simulink model "lev2coilsZpid"  (R2022a)
settings: Solver=ode3  StartTime=0.0  StopTime=5  FixedStep=1e-3  RelTol=1e-3
values from neighbouring files (symbols this model uses):
  g = s(1:n,n+1:n+nb)    [MagLev.m]    (also in MagLev4coils.m = 9.8)
  K3 = K1    (= 5.40205233157e-05)    [MagLev4coils.m]
  K4 = K2    (= 5.40205233157e-05)    [MagLev4coils.m]
  l = 0.0567/2    (= 0.02835)    [MagLev4coils.m]
  L1 = L    (= 0.00388)    [MagLev4coils.m]
  L2 = L    (= 0.00388)    [MagLev4coils.m]
  m = 0.03    [MagLev.m]    (also in MagLev4coils.m = 0.01)
  R1 = R    (= 4)    [MagLev4coils.m]
  R2 = R    (= 4)    [MagLev4coils.m]
settings Model: Creator=macbook_pro  LastModifiedBy=macbook_pro
settings DebuggingCC: UnconnectedInputMsg=warning  UnconnectedOutputMsg=warning  UnconnectedLineMsg=warning
settings RTWCC: DLArmComputeVersion=19.05

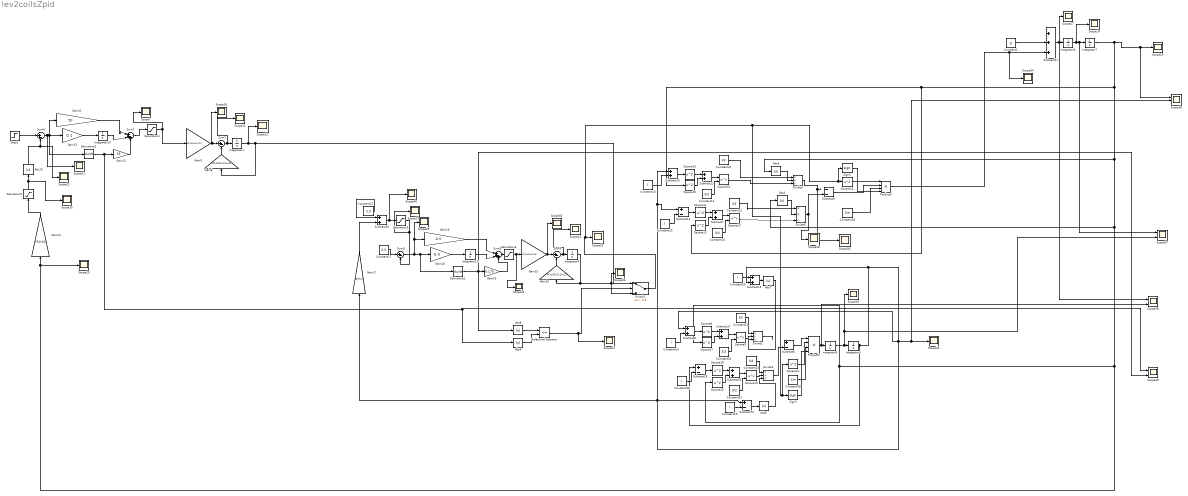
== system lev2coilsZpid ==
  Abs{4..10} (7 alike) : Abs  SaturateOnIntegerOverflow=off
  Constant1 : Constant  Value=g
  Constant11 : Constant  Value=K3
  Constant12 : Constant  Value=K4
  Constant{13,15,19..20,24,36} (6 alike) : Constant  Value=l
  Constant{14,16,34,37} (4 alike) : Constant  Value=3/2
  Constant17 : Constant  Value=2.5
  Constant18 : Constant  Value=1/m
  Constant21 : Constant  Value=K3
  Constant22 : Constant  Value=2.5
  Constant23 : Constant  Value=K4
  Constant38 : Constant  Value=1/m
  Derivative1 : Derivative
  Derivative2 : Derivative
  Divide1 : Product  Inputs=*/*
  Divide4 : Product  Inputs=*/*
  Divide5 : Product  Inputs=**/
  Divide6 : Product  Inputs=**/
  Gain10 : Gain  Gain=(R1+R2)/(L1+L2)
  Gain11 : Gain  Gain=50
  Gain12 : Gain  Gain=55
  Gain13 : Gain  Gain=0.1
  Gain14 : Gain  Gain=(5/0.04)
  Gain15 : Gain  Gain=12/((L2+L1)*5)
  Gain16 : Gain  Gain=0.175
  Gain17 : Gain  Gain=5/(l*2)
  Gain18 : Gain  Gain=0.5
  Gain19 : Gain  Gain=-0.5
  Gain8 : Gain  Gain=(R1+R2)/(L1+L2)
  Gain9 : Gain  Gain=12/((L2+L1)*5)
  Integrator{1,4,6,9..11} (6 alike) : Integrator
  Integrator5 : Integrator  InitialCondition=l
  Integrator7 : Integrator  InitialCondition=-0.03
  Product2 : Product  Inputs=4
  Product3 : Product  Inputs=4
  Relational Operator : RelationalOperator  Operator=<=  OutDataTypeStr=boolean  RndMeth=Simplest  InputSameDT=off
  Saturation3 : Saturate  UpperLimit=5  LowerLimit=0
  Saturation4 : Saturate  UpperLimit=5  LowerLimit=-5
  Saturation5 : Saturate  UpperLimit=0  LowerLimit=-5
  Saturation6 : Saturate  UpperLimit=5  LowerLimit=-5
  Scope{7,11..12,14,16..17,19..35,40..41} (25 alike) : Scope
  Scope36 : Scope  NumInputPorts=3
  Scope37 : Scope  NumInputPorts=2
  Scope38 : Scope  NumInputPorts=2
  Scope39 : Scope  NumInputPorts=2
  Sign2 : Signum
  Sign3 : Signum
  Square{8,10..11,13..15,17..18,20..21} (10 alike) : Math  Operator=square
  Square{9,12,16,19} (4 alike) : Math  Operator=pow
  Step1 : Step  Time=0  After=3.5  SampleTime=0
  Subtract{7..8,10,12,15..17,26} (8 alike) : Sum
  Subtract11 : Sum  Inputs=+++
  Subtract{6,13..14,18} (4 alike) : Sum  Inputs=+-
  Subtract9 : Sum  Inputs=--
  Sum{2..3,5..6} (4 alike) : Sum  Inputs=|+-
  Sum7 : Sum  Inputs=|+++
  Sum8 : Sum  Inputs=|+++
  Switch1 : Switch  Criteria=u2 > Threshold  Threshold=0.5  SaturateOnIntegerOverflow=off  InputSameDT=off
  wires:
  Gain8/1 -> Sum2/2
  Square9/1 -> Divide1/2
  Gain14/1 -> Saturation5/1
  Abs7/1 -> Divide1/3
  Constant19/1 -> Subtract14/2
  Gain9/1 -> Scope16/1, Sum2/1
  Abs6/1 -> Divide4/3
  Square18/1 -> Subtract26/1
  Sum7/1 -> Saturation4/1
  Constant13/1 -> Subtract10/2
  Subtract18/1 -> Square18/1
  Subtract11/1 -> Scope38/1, Scope17/1, Integrator6/1
  Sign3/1 -> Product2/4
  Square10/1 -> Subtract12/2
  Square13/1 -> Subtract7/2
  Constant36/1 -> Subtract18/2
  Step1/1 -> Sum6/1
  Square8/1 -> Subtract17/1
  Saturation4/1 -> Scope7/1, Gain9/1
  Divide1/1 -> ?
  Square16/1 -> Divide5/3
  Divide5/1 -> Scope30/1
  Divide4/1 -> Subtract6/2
  Abs4/1 -> Divide6/2
  Constant38/1 -> Product2/3
  Derivative2/1 -> Gain12/1, Abs9/1, Scope39/1
  Constant1/1 -> Subtract11/2
  Abs5/1 -> Divide5/2
  Constant12/1 -> Divide6/1
  Square11/1 -> Subtract7/1
  Sum3/1 -> Integrator4/1, Scope24/1
  Subtract12/1 -> Square16/1
  Switch1/1 -> Scope31/1, Square21/1, Sign3/1, Sign2/1, Square14/1
  Constant15/1 -> Subtract13/2
  Constant20/1 -> Subtract15/1
  Gain12/1 -> Sum7/3
  Subtract7/1 -> Square12/1
  Constant18/1 -> Product3/3
  Derivative1/1 -> Abs8/1, Gain16/1, Scope39/2
  Abs8/1 -> Relational Operator/1
  Constant37/1 -> Square19/2
  Integrator5/1 -> Subtract15/2, Subtract10/1, Subtract13/1, Gain17/1, Subtract14/1, Subtract8/1, Scope36/2, Scope23/1, Subtract18/1
  Integrator4/1 -> Scope26/1, Switch1/3, Gain10/1
  Abs9/1 -> Relational Operator/2
  Square21/1 -> Product2/2
  Product3/1 -> Scope34/1, Subtract11/3
  Subtract17/1 -> Square9/1
  Subtract26/1 -> Square19/1
  Subtract13/1 -> Square11/1
  Gain13/1 -> Integrator10/1
  Subtract15/1 -> Abs7/1
  Square20/1 -> Subtract26/2
  Gain15/1 -> Scope33/1, Sum3/1
  Integrator1/1 -> Scope12/1, Switch1/1, Gain8/1
  Integrator6/1 -> Scope37/1, Integrator7/1, Scope14/1
  Square12/1 -> Divide6/3
  Sum2/1 -> Scope11/1, Integrator1/1
  Square19/1 -> Divide4/2
  Subtract9/1 -> Product3/2
  Gain11/1 -> Sum7/1
  Abs10/1 -> Scope22/1, Sum6/2
  Sum6/1 -> Scope21/1, Derivative2/1, Gain13/1, Gain11/1
  Saturation5/1 -> Abs10/1, Scope35/1
  Sum8/1 -> Saturation6/1
  Subtract10/1 -> Square15/1
  Constant21/1 -> Divide5/1
  Square15/1 -> Subtract12/1
  Product2/1 -> Scope38/2, Integrator9/1
  Sum5/1 -> Gain19/1, Scope25/1, Derivative1/1, Gain18/1
  Gain18/1 -> Integrator11/1
  Divide6/1 -> Scope28/1, Subtract9/2
  Subtract8/1 -> Square8/1
  Sign2/1 -> Product3/4
  Gain16/1 -> Sum8/3
  Integrator7/1 -> Abs5/1, Abs4/1, Square17/1, Square20/1, Gain14/1, Scope20/1, Square13/1, Square10/1, Scope36/1, Scope19/1
  Gain19/1 -> Sum8/1
  Constant34/1 -> Square9/2
  Relational Operator/1 -> Scope41/1, Switch1/2
  Gain17/1 -> Subtract16/2
  Square14/1 -> Product3/1
  Subtract14/1 -> Abs6/1
  Constant17/1 -> Sum5/1
  Saturation3/1 -> Sum5/2, Scope27/1
  Integrator9/1 -> Scope37/2, Scope29/1, Integrator5/1
  Constant24/1 -> Subtract8/2
  Integrator11/1 -> Sum8/2
  Constant23/1 -> Divide4/1
  Subtract16/1 -> Scope40/1, Saturation3/1
  Gain10/1 -> Sum3/2
  Constant11/1 -> Divide1/1
  Saturation6/1 -> Scope32/1, Gain15/1
  Subtract6/1 -> Product2/1
  Constant14/1 -> Square16/2
  Constant22/1 -> Subtract16/1
  Square17/1 -> Subtract17/2
  Integrator10/1 -> Sum7/2
  Constant16/1 -> Square12/2
